simulink model "simINVD_ssm"  (R2021b)
settings: Solver=FixedStepAuto  StartTime=0.0  StopTime=simTime  FixedStep=stepSize
values from neighbouring files (symbols this model uses):
  drv1 = Transmission    [sd_ssm.m]
  drv2 = Transmission    [sd_ssm.m]
  drv4 = Transmission    [sd_ssm.m]
  initConfig = [0 0 0 0]    [ssmMotorization.m]
  jointIdx = 2    [ssmMotorization.m]
  maxAccel = 10    [ssmMotorization.m]
  maxVel = 2    [ssmMotorization.m]
  timeStamps = [t1 t2 t3 t4 t5 t6 t7 t8 t9 t10 t11 t12]    [ssmMotorization.m]
libraries: robotmaniplib x4
settings Model: Creator=anestis  LastModifiedBy=Anestis Mablekos
settings SolverCC: AlgebraicLoopSolver=TrustRegion  SolverResetMethod=Robust
settings DataIOCC: ReturnWorkspaceOutputs=off
settings DebuggingCC: SFMachineParentedDataDiag=warning  ArithmeticOperatorsInVariantConditions=warning
settings SFSimCC: SimUseLocalCustomCode=off  CustomCodeUndefinedFunction=UseInterfaceOnly
settings RTWCC: RTWUseLocalCustomCode=off
settings CodeAppCC: StateflowObjectComments=on

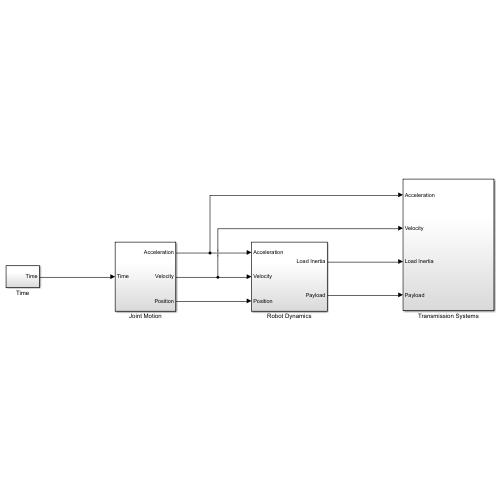
[thumbnail: Simulink's stored preview of the top-level diagram]
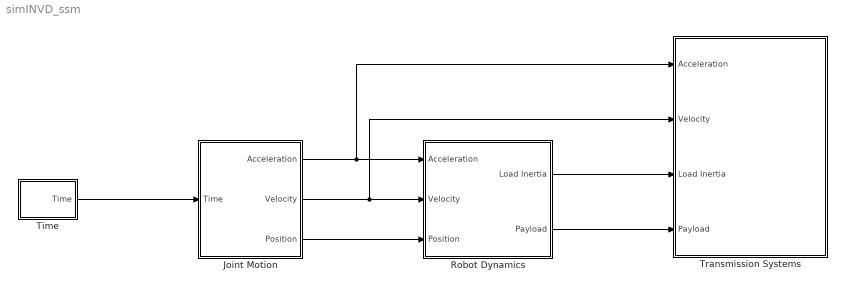
== system simINVD_ssm ==
  Joint Motion : Subsystem
  Robot Dynamics : Subsystem
  Time : Subsystem
  Transmission Systems : Subsystem
  wires:
  Robot Dynamics/1(Load Inertia) -> Transmission Systems/3(Load Inertia)
  Robot Dynamics/2(Payload) -> Transmission Systems/4(Payload)
  Time/1(Time) -> Joint Motion/1(Time)
  Joint Motion/1(Acceleration) -> Transmission Systems/1(Acceleration), Robot Dynamics/1(Acceleration)
  Joint Motion/2(Velocity) -> Robot Dynamics/2(Velocity), Transmission Systems/2(Velocity)
  Joint Motion/3(Position) -> Robot Dynamics/3(Position)

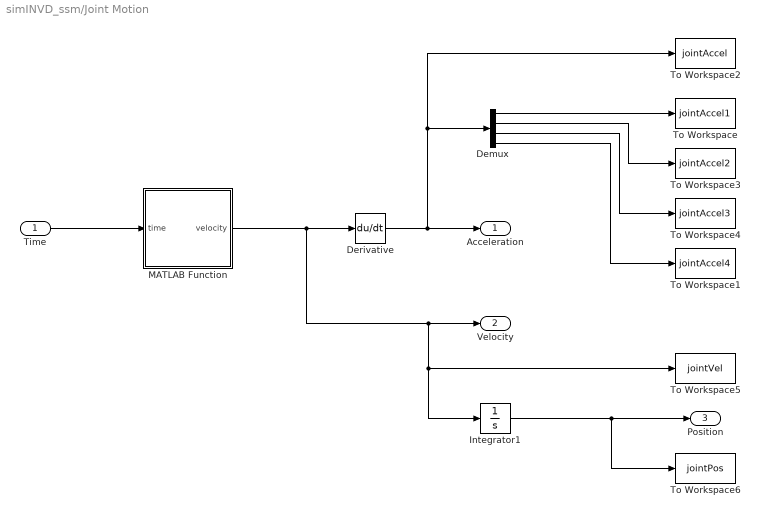
== system simINVD_ssm/Joint Motion ==
  Time : Inport
  Demux : Demux
  Derivative : Derivative
  Integrator1 : Integrator  InitialCondition=initConfig
  MATLAB Function : MATLAB Function  TreatAsAtomicUnit=on
  To Workspace : ToWorkspace  VariableName=jointAccel1  SaveFormat=Timeseries  SampleTime=-1
  To Workspace1 : ToWorkspace  VariableName=jointAccel4  SaveFormat=Timeseries  SampleTime=-1
  To Workspace2 : ToWorkspace  VariableName=jointAccel  SaveFormat=Timeseries  SampleTime=-1
  To Workspace3 : ToWorkspace  VariableName=jointAccel2  SaveFormat=Timeseries  SampleTime=-1
  To Workspace4 : ToWorkspace  VariableName=jointAccel3  SaveFormat=Timeseries  SampleTime=-1
  To Workspace5 : ToWorkspace  VariableName=jointVel  SaveFormat=Timeseries  SampleTime=-1
  To Workspace6 : ToWorkspace  VariableName=jointPos  SaveFormat=Timeseries  SampleTime=-1
  Acceleration : Outport
  Velocity : Outport  Port=2
  Position : Outport  Port=3
  wires:
  Time/1 -> MATLAB Function/1(time)
  Demux/1 -> To Workspace/1
  Demux/4 -> To Workspace1/1
  Demux/2 -> To Workspace3/1
  Demux/3 -> To Workspace4/1
  MATLAB Function/1(velocity) -> Velocity/1, To Workspace5/1, Integrator1/1, Derivative/1
  Integrator1/1 -> To Workspace6/1, Position/1
  Derivative/1 -> Demux/1, To Workspace2/1, Acceleration/1

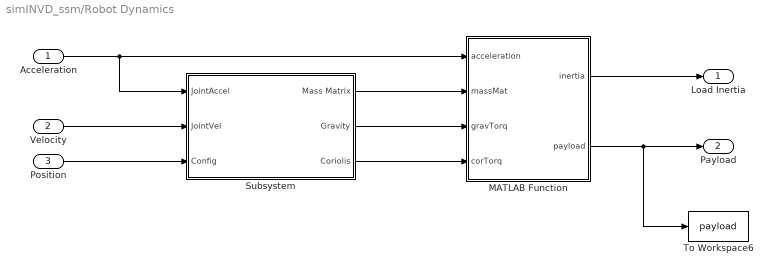
== system simINVD_ssm/Robot Dynamics ==
  Acceleration : Inport
  Velocity : Inport  Port=2
  Position : Inport  Port=3
  MATLAB Function : MATLAB Function  TreatAsAtomicUnit=on
  Subsystem : Subsystem
  To Workspace6 : ToWorkspace  VariableName=payload  SaveFormat=Timeseries  SampleTime=-1
  Load Inertia : Outport
  Payload : Outport  Port=2
  wires:
  Velocity/1 -> Subsystem/2(JointVel)
  Position/1 -> Subsystem/3(Config)
  Subsystem/2(Gravity) -> MATLAB Function/3(gravTorq)
  Subsystem/1(Mass Matrix) -> MATLAB Function/2(massMat)
  Subsystem/3(Coriolis) -> MATLAB Function/4(corTorq)
  Acceleration/1 -> Subsystem/1(JointAccel), MATLAB Function/1(acceleration)
  MATLAB Function/1(inertia) -> Load Inertia/1
  MATLAB Function/2(payload) -> To Workspace6/1, Payload/1

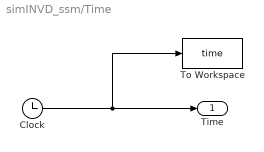
== system simINVD_ssm/Time ==
  Clock : Clock
  To Workspace : ToWorkspace  VariableName=time  SaveFormat=Timeseries  SampleTime=-1
  Time : Outport
  wires:
  Clock/1 -> Time/1, To Workspace/1

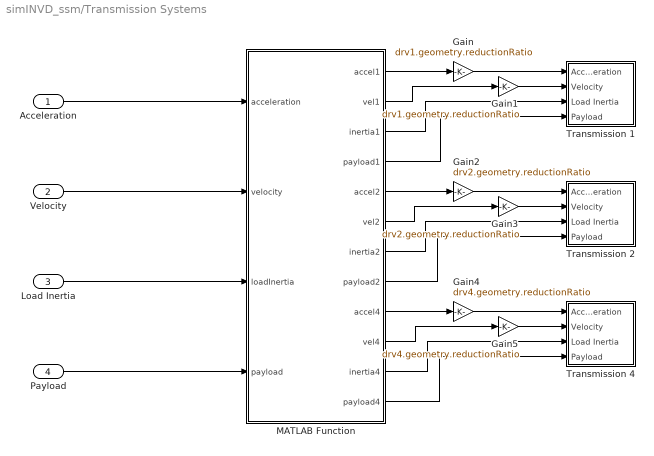
== system simINVD_ssm/Transmission Systems ==
  Acceleration : Inport
  Velocity : Inport  Port=2
  Load Inertia : Inport  Port=3
  Payload : Inport  Port=4
  Gain : Gain  Gain=drv1.geometry.reductionRatio
  Gain1 : Gain  Gain=drv1.geometry.reductionRatio
  Gain2 : Gain  Gain=drv2.geometry.reductionRatio
  Gain3 : Gain  Gain=drv2.geometry.reductionRatio
  Gain4 : Gain  Gain=drv4.geometry.reductionRatio
  Gain5 : Gain  Gain=drv4.geometry.reductionRatio
  MATLAB Function : MATLAB Function  TreatAsAtomicUnit=on
  Transmission 1 : Subsystem
  Transmission 2 : Subsystem
  Transmission 4 : Subsystem
  wires:
  MATLAB Function/3(inertia1) -> Transmission 1/3(Load Inertia)
  MATLAB Function/4(payload1) -> Transmission 1/4(Payload)
  Velocity/1 -> MATLAB Function/2(velocity)
  Load Inertia/1 -> MATLAB Function/3(loadInertia)
  Payload/1 -> MATLAB Function/4(payload)
  Acceleration/1 -> MATLAB Function/1(acceleration)
  MATLAB Function/12(payload4) -> Transmission 4/4(Payload)
  MATLAB Function/11(inertia4) -> Transmission 4/3(Load Inertia)
  MATLAB Function/10(vel4) -> Gain5/1
  MATLAB Function/9(accel4) -> Gain4/1
  MATLAB Function/8(payload2) -> Transmission 2/4(Payload)
  MATLAB Function/7(inertia2) -> Transmission 2/3(Load Inertia)
  MATLAB Function/6(vel2) -> Gain3/1
  MATLAB Function/5(accel2) -> Gain2/1
  MATLAB Function/1(accel1) -> Gain/1
  MATLAB Function/2(vel1) -> Gain1/1
  Gain/1 -> Transmission 1/1(Acceleration)
  Gain1/1 -> Transmission 1/2(Velocity)
  Gain2/1 -> Transmission 2/1(Acceleration)
  Gain3/1 -> Transmission 2/2(Velocity)
  Gain4/1 -> Transmission 4/1(Acceleration)
  Gain5/1 -> Transmission 4/2(Velocity)

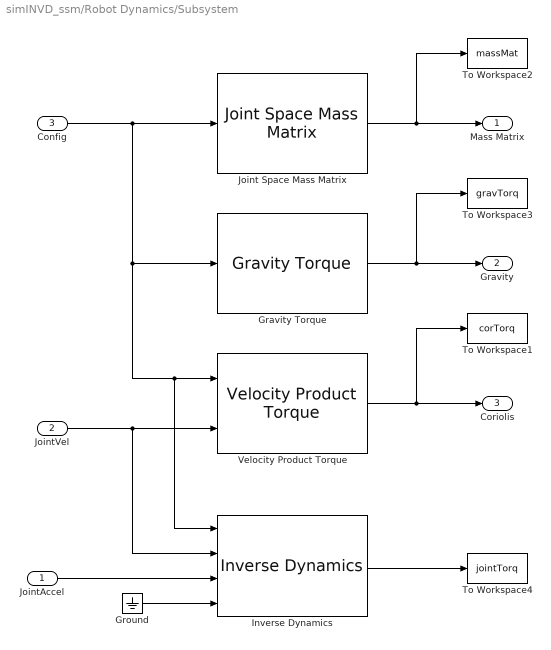
== system simINVD_ssm/Robot Dynamics/Subsystem ==
  JointAccel : Inport
  JointVel : Inport  Port=2
  Config : Inport  Port=3
  Gravity Torque : robotmaniplib/Gravity Torque  RigidBodyTree=robot  SimulateUsing=Interpreted execution
  Ground : Ground
  Inverse Dynamics : robotmaniplib/Inverse Dynamics  RigidBodyTree=robot  SimulateUsing=Interpreted execution
      settings: SourceProductBaseCode=RO
  Joint Space Mass Matrix : robotmaniplib/Joint Space Mass Matrix  RigidBodyTree=robot  SimulateUsing=Interpreted execution
  To Workspace1 : ToWorkspace  VariableName=corTorq  SaveFormat=Timeseries  SampleTime=-1
  To Workspace2 : ToWorkspace  VariableName=massMat  SaveFormat=Timeseries  SampleTime=-1
  To Workspace3 : ToWorkspace  VariableName=gravTorq  SaveFormat=Timeseries  SampleTime=-1
  To Workspace4 : ToWorkspace  VariableName=jointTorq  SaveFormat=Timeseries  SampleTime=-1
  Velocity Product Torque : robotmaniplib/Velocity Product Torque  RigidBodyTree=robot  SimulateUsing=Interpreted execution
      settings: SourceProductBaseCode=RO
  Mass Matrix : Outport
  Gravity : Outport  Port=2
  Coriolis : Outport  Port=3
  wires:
  Config/1 -> Joint Space Mass Matrix/1, Inverse Dynamics/1, Velocity Product Torque/1, Gravity Torque/1
  JointVel/1 -> Inverse Dynamics/2, Velocity Product Torque/2
  Joint Space Mass Matrix/1 -> Mass Matrix/1, To Workspace2/1
  Gravity Torque/1 -> Gravity/1, To Workspace3/1
  Velocity Product Torque/1 -> To Workspace1/1, Coriolis/1
  JointAccel/1 -> Inverse Dynamics/3
  Ground/1 -> Inverse Dynamics/4
  Inverse Dynamics/1 -> To Workspace4/1

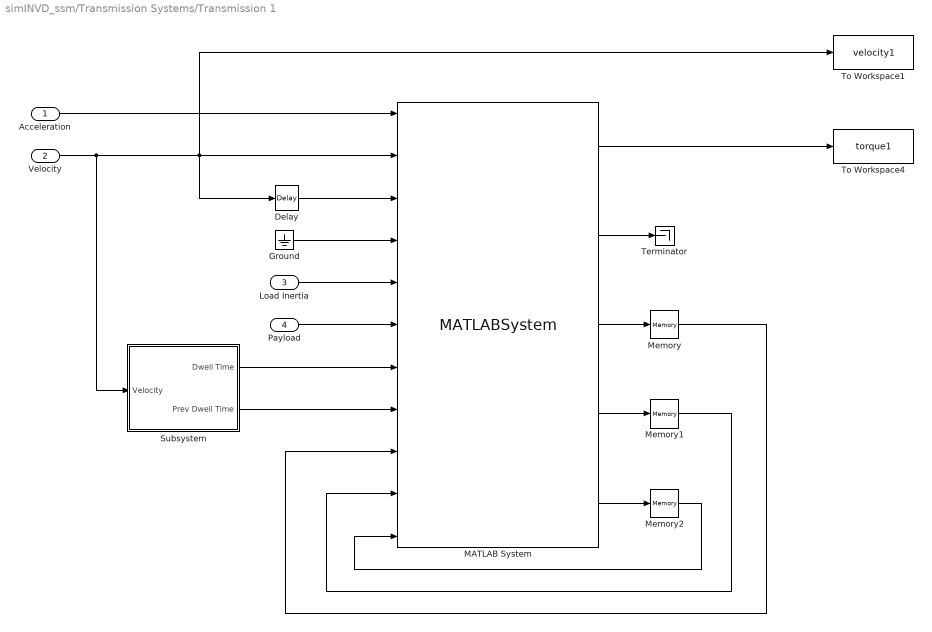
== system simINVD_ssm/Transmission Systems/Transmission 1 ==
  Acceleration : Inport
  Velocity : Inport  Port=2
  Load Inertia : Inport  Port=3
  Payload : Inport  Port=4
  Delay : TransportDelay  DelayTime=drv1.friction.memoryCst
  Ground : Ground
  MATLAB System : MATLABSystem  System=Transmission  geometry=drv1.geometry  preload=drv1.preload  friction=drv1.friction  inertia=drv1.inertia  actuation=drv1.actuation  SimulateUsing=Code generation
      mask Type: Transmission
      mask Display:
      | disp('Transmission');
      | port_label('input',1,'acceleration');
      | port_label('input',2,'velocity');
      | port_label('input',3,'velocityD');
      | port_label('input',4,'actrTorque');
      | port_label('input',5,'loadInertia');
      | port_label('input',6,'payload');
      | port_label('input',7,'dwellTime');
      | port_label('input',8,'dwellTimePrev');
      | port_label('input',9,'frictionCoeffPrev');
      | port_label('input',10,'strbFrictionPrev');
      | port_label('input',11,'strbArrivalPrev');
      | port_label('output',1,'torque');
      | port_label('output',2,'acceleration');
      | port_label('output',3,'frictionCoeff');
      | port_label('output',4,'strbFriction');
      | port_label('output',5,'strbArrival');
  Memory : Memory  InitialCondition=drv1.friction.strbInf + drv1.friction.kinFriction
  Memory1 : Memory  InitialCondition=drv1.friction.strbInf  InheritSampleTime=on
  Memory2 : Memory  InitialCondition=drv1.friction.strbInf
  Subsystem : Subsystem
  Terminator : Terminator
  To Workspace1 : ToWorkspace  VariableName=velocity1  SaveFormat=Timeseries  SampleTime=-1
  To Workspace4 : ToWorkspace  VariableName=torque1  SaveFormat=Timeseries  SampleTime=-1
  wires:
  Memory/1 -> MATLAB System/9
  Payload/1 -> MATLAB System/6
  Load Inertia/1 -> MATLAB System/5
  Memory1/1 -> MATLAB System/10
  Ground/1 -> MATLAB System/4
  Subsystem/2(Prev Dwell Time) -> MATLAB System/8
  Subsystem/1(Dwell Time) -> MATLAB System/7
  Memory2/1 -> MATLAB System/11
  MATLAB System/1 -> To Workspace4/1
  MATLAB System/2 -> Terminator/1
  Delay/1 -> MATLAB System/3
  MATLAB System/5 -> Memory2/1
  MATLAB System/3 -> Memory/1
  MATLAB System/4 -> Memory1/1
  Acceleration/1 -> MATLAB System/1
  Velocity/1 -> Subsystem/1(Velocity), To Workspace1/1, Delay/1, MATLAB System/2

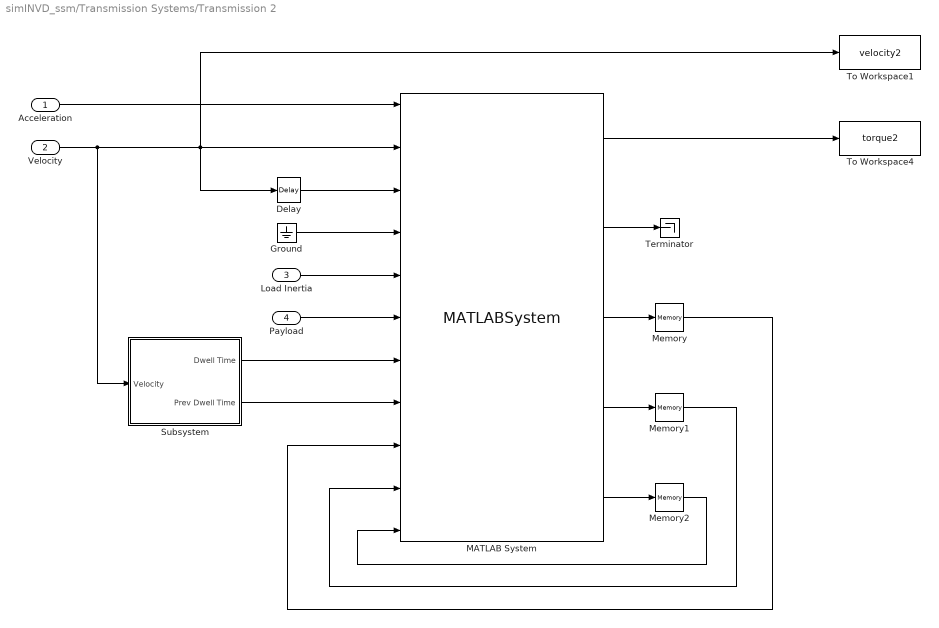
== system simINVD_ssm/Transmission Systems/Transmission 2 ==
  Acceleration : Inport
  Velocity : Inport  Port=2
  Load Inertia : Inport  Port=3
  Payload : Inport  Port=4
  Delay : TransportDelay  DelayTime=drv2.friction.memoryCst
  Ground : Ground
  MATLAB System : MATLABSystem  System=Transmission  geometry=drv2.geometry  preload=drv2.preload  friction=drv2.friction  inertia=drv2.inertia  actuation=drv2.actuation  SimulateUsing=Code generation
      mask Type: Transmission
      mask Display:
      | disp('Transmission');
      | port_label('input',1,'acceleration');
      | port_label('input',2,'velocity');
      | port_label('input',3,'velocityD');
      | port_label('input',4,'actrTorque');
      | port_label('input',5,'loadInertia');
      | port_label('input',6,'payload');
      | port_label('input',7,'dwellTime');
      | port_label('input',8,'dwellTimePrev');
      | port_label('input',9,'frictionCoeffPrev');
      | port_label('input',10,'strbFrictionPrev');
      | port_label('input',11,'strbArrivalPrev');
      | port_label('output',1,'torque');
      | port_label('output',2,'acceleration');
      | port_label('output',3,'frictionCoeff');
      | port_label('output',4,'strbFriction');
      | port_label('output',5,'strbArrival');
  Memory : Memory  InitialCondition=drv2.friction.strbInf + drv2.friction.kinFriction
  Memory1 : Memory  InitialCondition=drv2.friction.strbInf  InheritSampleTime=on
  Memory2 : Memory  InitialCondition=drv2.friction.strbInf
  Subsystem : Subsystem
  Terminator : Terminator
  To Workspace1 : ToWorkspace  VariableName=velocity2  SaveFormat=Timeseries  SampleTime=-1
  To Workspace4 : ToWorkspace  VariableName=torque2  SaveFormat=Timeseries  SampleTime=-1
  wires:
  Memory/1 -> MATLAB System/9
  Payload/1 -> MATLAB System/6
  Load Inertia/1 -> MATLAB System/5
  Memory1/1 -> MATLAB System/10
  Ground/1 -> MATLAB System/4
  Subsystem/2(Prev Dwell Time) -> MATLAB System/8
  Subsystem/1(Dwell Time) -> MATLAB System/7
  Memory2/1 -> MATLAB System/11
  MATLAB System/1 -> To Workspace4/1
  MATLAB System/2 -> Terminator/1
  Delay/1 -> MATLAB System/3
  MATLAB System/5 -> Memory2/1
  MATLAB System/3 -> Memory/1
  MATLAB System/4 -> Memory1/1
  Acceleration/1 -> MATLAB System/1
  Velocity/1 -> Subsystem/1(Velocity), To Workspace1/1, Delay/1, MATLAB System/2

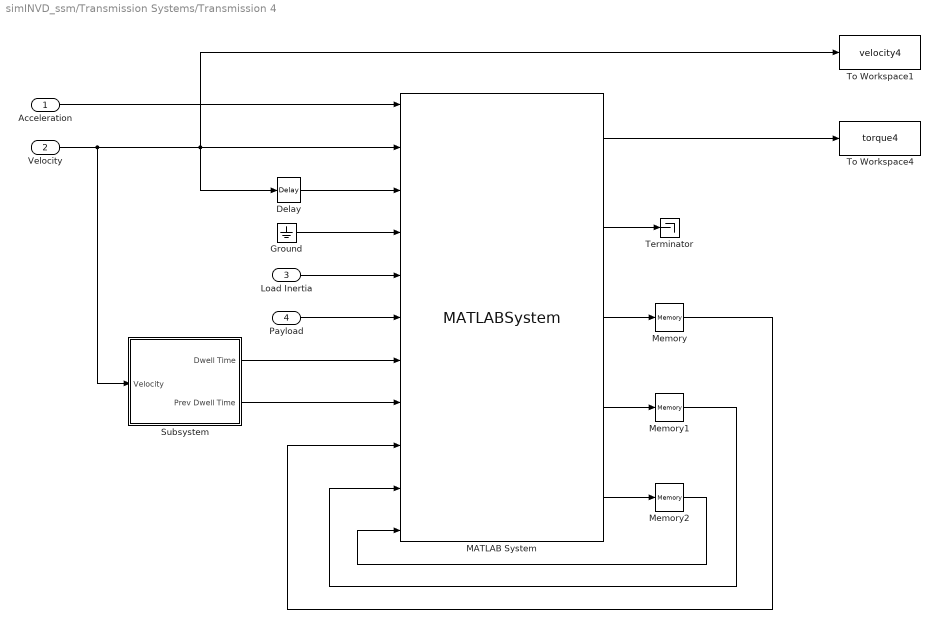
== system simINVD_ssm/Transmission Systems/Transmission 4 ==
  Acceleration : Inport
  Velocity : Inport  Port=2
  Load Inertia : Inport  Port=3
  Payload : Inport  Port=4
  Delay : TransportDelay  DelayTime=drv4.friction.memoryCst
  Ground : Ground
  MATLAB System : MATLABSystem  System=Transmission  geometry=drv4.geometry  preload=drv4.preload  friction=drv4.friction  inertia=drv4.inertia  actuation=drv4.actuation  SimulateUsing=Code generation
      mask Type: Transmission
      mask Display:
      | disp('Transmission');
      | port_label('input',1,'acceleration');
      | port_label('input',2,'velocity');
      | port_label('input',3,'velocityD');
      | port_label('input',4,'actrTorque');
      | port_label('input',5,'loadInertia');
      | port_label('input',6,'payload');
      | port_label('input',7,'dwellTime');
      | port_label('input',8,'dwellTimePrev');
      | port_label('input',9,'frictionCoeffPrev');
      | port_label('input',10,'strbFrictionPrev');
      | port_label('input',11,'strbArrivalPrev');
      | port_label('output',1,'torque');
      | port_label('output',2,'acceleration');
      | port_label('output',3,'frictionCoeff');
      | port_label('output',4,'strbFriction');
      | port_label('output',5,'strbArrival');
  Memory : Memory  InitialCondition=drv4.friction.strbInf + drv4.friction.kinFriction
  Memory1 : Memory  InitialCondition=drv4.friction.strbInf  InheritSampleTime=on
  Memory2 : Memory  InitialCondition=drv4.friction.strbInf
  Subsystem : Subsystem
  Terminator : Terminator
  To Workspace1 : ToWorkspace  VariableName=velocity4  SaveFormat=Timeseries  SampleTime=-1
  To Workspace4 : ToWorkspace  VariableName=torque4  SaveFormat=Timeseries  SampleTime=-1
  wires:
  Memory/1 -> MATLAB System/9
  Payload/1 -> MATLAB System/6
  Load Inertia/1 -> MATLAB System/5
  Memory1/1 -> MATLAB System/10
  Ground/1 -> MATLAB System/4
  Subsystem/2(Prev Dwell Time) -> MATLAB System/8
  Subsystem/1(Dwell Time) -> MATLAB System/7
  Memory2/1 -> MATLAB System/11
  MATLAB System/1 -> To Workspace4/1
  MATLAB System/2 -> Terminator/1
  Delay/1 -> MATLAB System/3
  MATLAB System/5 -> Memory2/1
  MATLAB System/3 -> Memory/1
  MATLAB System/4 -> Memory1/1
  Acceleration/1 -> MATLAB System/1
  Velocity/1 -> Subsystem/1(Velocity), To Workspace1/1, Delay/1, MATLAB System/2

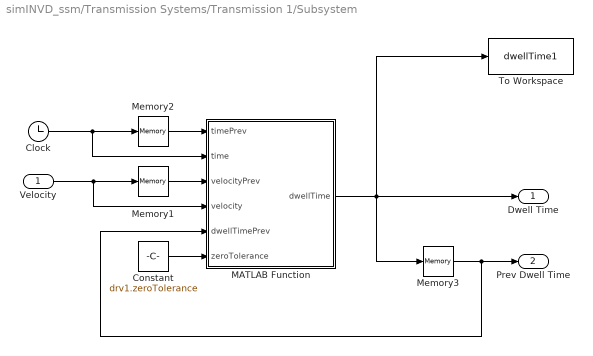
== system simINVD_ssm/Transmission Systems/Transmission 1/Subsystem ==
  Velocity : Inport
  Clock : Clock
  Constant : Constant  Value=drv1.zeroTolerance
  MATLAB Function : MATLAB Function  TreatAsAtomicUnit=on
  Memory1 : Memory
  Memory2 : Memory
  Memory3 : Memory  InitialCondition=100  LinearizeMemory=on
  To Workspace : ToWorkspace  VariableName=dwellTime1  SaveFormat=Timeseries  SampleTime=-1
  Dwell Time : Outport
  Prev Dwell Time : Outport  Port=2
  wires:
  MATLAB Function/1(dwellTime) -> To Workspace/1, Dwell Time/1, Memory3/1
  Clock/1 -> MATLAB Function/2(time), Memory2/1
  Velocity/1 -> MATLAB Function/4(velocity), Memory1/1
  Memory3/1 -> MATLAB Function/5(dwellTimePrev), Prev Dwell Time/1
  Constant/1 -> MATLAB Function/6(zeroTolerance)
  Memory2/1 -> MATLAB Function/1(timePrev)
  Memory1/1 -> MATLAB Function/3(velocityPrev)

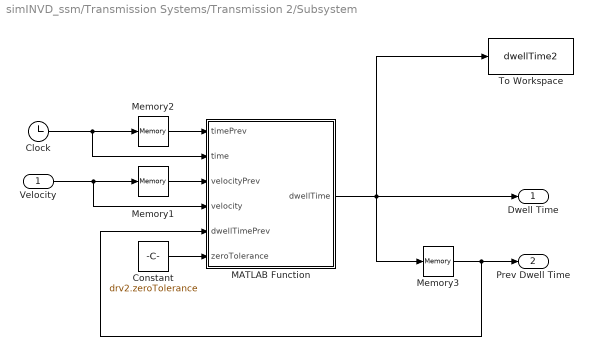
== system simINVD_ssm/Transmission Systems/Transmission 2/Subsystem ==
  Velocity : Inport
  Clock : Clock
  Constant : Constant  Value=drv2.zeroTolerance
  MATLAB Function : MATLAB Function  TreatAsAtomicUnit=on
  Memory1 : Memory
  Memory2 : Memory
  Memory3 : Memory  InitialCondition=100  LinearizeMemory=on
  To Workspace : ToWorkspace  VariableName=dwellTime2  SaveFormat=Timeseries  SampleTime=-1
  Dwell Time : Outport
  Prev Dwell Time : Outport  Port=2
  wires:
  MATLAB Function/1(dwellTime) -> To Workspace/1, Dwell Time/1, Memory3/1
  Clock/1 -> MATLAB Function/2(time), Memory2/1
  Velocity/1 -> MATLAB Function/4(velocity), Memory1/1
  Memory3/1 -> MATLAB Function/5(dwellTimePrev), Prev Dwell Time/1
  Constant/1 -> MATLAB Function/6(zeroTolerance)
  Memory2/1 -> MATLAB Function/1(timePrev)
  Memory1/1 -> MATLAB Function/3(velocityPrev)

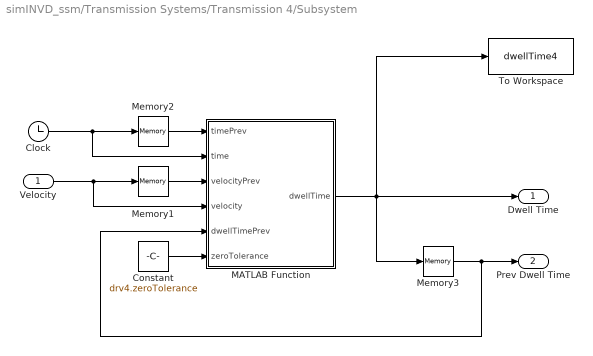
== system simINVD_ssm/Transmission Systems/Transmission 4/Subsystem ==
  Velocity : Inport
  Clock : Clock
  Constant : Constant  Value=drv4.zeroTolerance
  MATLAB Function : MATLAB Function  TreatAsAtomicUnit=on
  Memory1 : Memory
  Memory2 : Memory
  Memory3 : Memory  InitialCondition=100  LinearizeMemory=on
  To Workspace : ToWorkspace  VariableName=dwellTime4  SaveFormat=Timeseries  SampleTime=-1
  Dwell Time : Outport
  Prev Dwell Time : Outport  Port=2
  wires:
  MATLAB Function/1(dwellTime) -> To Workspace/1, Dwell Time/1, Memory3/1
  Clock/1 -> MATLAB Function/2(time), Memory2/1
  Velocity/1 -> MATLAB Function/4(velocity), Memory1/1
  Memory3/1 -> MATLAB Function/5(dwellTimePrev), Prev Dwell Time/1
  Constant/1 -> MATLAB Function/6(zeroTolerance)
  Memory2/1 -> MATLAB Function/1(timePrev)
  Memory1/1 -> MATLAB Function/3(velocityPrev)

== matlab function simINVD_ssm/Joint Motion/MATLAB Function ==
  data: time input; velocity output; timeStamps parameter; maxAccel parameter; maxVel parameter; jointIdx parameter
function velocity = fcn(time, timeStamps, maxAccel, maxVel, jointIdx)

velocity = zeros(4,1);

if time <= timeStamps(1)
    jointVel = 0;
elseif time > timeStamps(1) && time <= timeStamps(2)
    jointVel = maxAccel*(time-timeStamps(1));
elseif time > timeStamps(2) && time <= timeStamps(3)
    jointVel = maxVel;
elseif time > timeStamps(3) && time <= timeStamps(4)
    jointVel = maxVel-maxAccel*(time-timeStamps(3));
elseif time > timeStamps(4) && time <= timeStamps(5)
    jointVel = -maxVel;
elseif time > timeStamps(5) && time <= timeStamps(6)
    jointVel = -maxVel+maxAccel*(time-timeStamps(5));
elseif time > timeStamps(6) && time <= timeStamps(7)
    jointVel = 0;
elseif time > timeStamps(7) && time <= timeStamps(8)
    jointVel = -maxAccel*(time-timeStamps(7));
elseif time > timeStamps(8) && time <= timeStamps(9)
    jointVel = -maxVel;
elseif time > timeStamps(9) && time <= timeStamps(10)
    jointVel = -maxVel+maxAccel*(time-timeStamps(9));
elseif time > timeStamps(10) && time <= timeStamps(11)
    jointVel = maxVel;
elseif time > timeStamps(11) && time <= timeStamps(12)
    jointVel = maxVel-maxAccel*(time-timeStamps(11));
else
    jointVel = 0;
end

velocity(jointIdx) = jointVel;

end

== matlab function simINVD_ssm/Transmission Systems/Transmission 1/Subsystem/MATLAB Function ==
  data: timePrev input; time input; velocityPrev input; velocity input; dwellTime output; dwellTimePrev input; zeroTolerance input
function dwellTime = fcn(timePrev, time, velocityPrev, velocity, dwellTimePrev, zeroTolerance)

int = time-timePrev;

if abs(velocity) < zeroTolerance
    if abs(velocity-velocityPrev) < zeroTolerance
        dwellTime = int + dwellTimePrev;
    else
        dwellTime = 0;
    end
else
    dwellTime = 0;
end

== matlab function simINVD_ssm/Robot Dynamics/MATLAB Function ==
  data: acceleration input; massMat input; inertia output; gravTorq input; corTorq input; payload output
function [inertia, payload] = fcn(acceleration, massMat, gravTorq, corTorq)


inertia = diag(massMat);
inertiaTorq = (massMat - diag(diag(massMat)))*acceleration;
payload = -(inertiaTorq + gravTorq - corTorq);

== matlab function simINVD_ssm/Transmission Systems/Transmission 2/Subsystem/MATLAB Function ==
  data: timePrev input; time input; velocityPrev input; velocity input; dwellTime output; dwellTimePrev input; zeroTolerance input
function dwellTime = fcn(timePrev, time, velocityPrev, velocity, dwellTimePrev, zeroTolerance)

int = time-timePrev;

if abs(velocity) < zeroTolerance
    if abs(velocity-velocityPrev) < zeroTolerance
        dwellTime = int + dwellTimePrev;
    else
        dwellTime = 0;
    end
else
    dwellTime = 0;
end

== matlab function simINVD_ssm/Transmission Systems/MATLAB Function ==
  data: acceleration input; velocity input; accel1 output; loadInertia input; payload input; vel1 output; inertia1 output; payload1 output; accel2 output; vel2 output; inertia2 output; payload2 output; accel4 output; vel4 output; inertia4 output; payload4 output
function [accel1, vel1, inertia1, payload1,...
    accel2, vel2, inertia2, payload2,...
    accel4, vel4, inertia4, payload4] = fcn(acceleration, velocity, loadInertia, payload)

accel1 = acceleration(1);
vel1 = velocity(1);
inertia1 = loadInertia(1);
payload1 = payload(1);

accel2 = acceleration(2);
vel2 = velocity(2);
inertia2 = loadInertia(2);
payload2 = payload(2);

accel4 = acceleration(4);
vel4 = velocity(4);
inertia4 = loadInertia(4);
payload4 = payload(4);

== matlab function simINVD_ssm/Transmission Systems/Transmission 4/Subsystem/MATLAB Function ==
  data: timePrev input; time input; velocityPrev input; velocity input; dwellTime output; dwellTimePrev input; zeroTolerance input
function dwellTime = fcn(timePrev, time, velocityPrev, velocity, dwellTimePrev, zeroTolerance)

int = time-timePrev;

if abs(velocity) < zeroTolerance
    if abs(velocity-velocityPrev) < zeroTolerance
        dwellTime = int + dwellTimePrev;
    else
        dwellTime = 0;
    end
else
    dwellTime = 0;
end
